simulink model "CuantUnifSin"  (R2014a)
settings: Solver=ode45  StartTime=0.0  StopTime=10.0  RelTol=1e-3
values from neighbouring files (symbols this model uses):
  n = N(i)    [CuantNoUniformeVoz.m]    (also in CuantUniformeSeno.m; CuantUniformeVoz.m)
settings Model: Creator=Jorge Armando  LastModifiedBy=joshue
settings DataIOCC: LimitDataPoints=off
settings DebuggingCC: UnderspecifiedInitializationDetection=Classic  StateNameClashWarn=warning

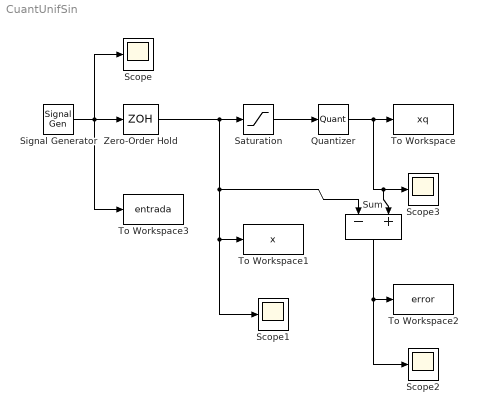
== system CuantUnifSin ==
  Quantizer : Quantizer  QuantizationInterval=2^(1-n)
  Saturation : Saturate  UpperLimit=1  LowerLimit=-1
  Scope{,1..3} (4 alike) : Scope
      Scope2 settings: SaveName=ScopeData2
      Scope3 settings: SaveName=ScopeData3
  Signal Generator : SignalGenerator
  Sum : Sum  Inputs=|-+
  To Workspace : ToWorkspace  VariableName=xq  SampleTime=-1
  To Workspace1 : ToWorkspace  VariableName=x  SampleTime=-1
  To Workspace2 : ToWorkspace  VariableName=error  SampleTime=-1
  To Workspace3 : ToWorkspace  VariableName=entrada  SampleTime=-1
  Zero-Order Hold : ZeroOrderHold  SampleTime=.01
  wires:
  Signal Generator/1 -> To Workspace3/1, Scope/1, Zero-Order Hold/1
  Zero-Order Hold/1 -> Scope1/1, To Workspace1/1, Sum/1, Saturation/1
  Saturation/1 -> Quantizer/1
  Quantizer/1 -> Scope3/1, Sum/2, To Workspace/1
  Sum/1 -> Scope2/1, To Workspace2/1
